simulink model "TransmissionSystem"  (R2026a)
settings: Solver=FixedStepAuto  StopTime=65  FixedStep=0.0005
undefined symbols (not defined in the file or in its folder): f3ea6d5f
settings Model: DataDictionary=ETRS_data.sldd  VariantConfigurationObject=vConfigData  Creator=macec  LastModifiedBy=tstic

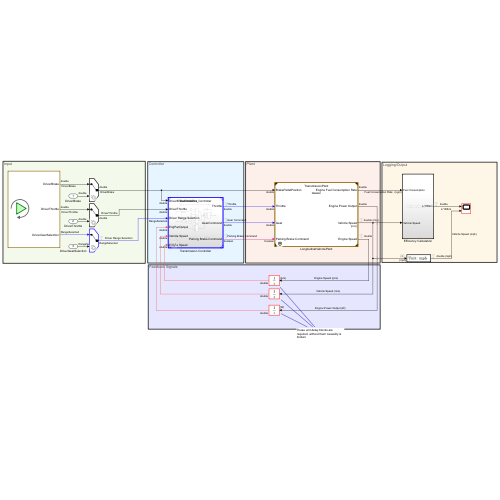
[thumbnail: Simulink's stored preview of the top-level diagram]
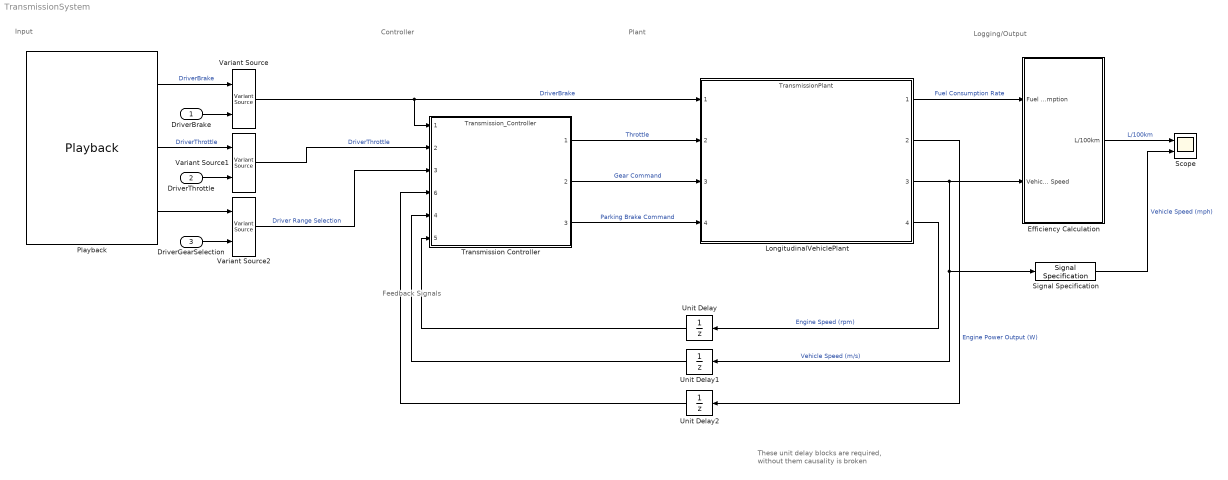
== system TransmissionSystem ==
  note: Logging/Output
  note: These unit delay blocks are required, without them causality is broken
  note: Feedback Signals
  note: Plant
  note: Controller
  note: Input
  DriverBrake : Inport  Interpolate=off
  DriverThrottle : Inport  Port=2  Interpolate=off
  DriverGearSelection : Inport  Port=3  OutDataTypeStr=Enum: RangeSelected  Interpolate=off
  Efficiency Calculation : Subsystem
  LongitudinalVehiclePlant : ModelReference  ModelNameDialog=TransmissionPlant.slxp  ModelReferenceVersion=1.92  CopyOfModelProtected=on  InputSignalHandling=Zero-order hold
  Playback : Playback  NumPorts=3  PartName=f3ea6d5f-6941-4fcc-8b84-64e5b7c9aa8d  TablePosition=Bottom
  Scope : Scope  NumInputPorts=2
  Signal Specification : SignalSpecification  Unit=mph
  Transmission Controller : ModelReference  ModelNameDialog=Transmission_Controller  SimulationMode=Normal  ModelReferenceVersion=1.50
      settings: PortSchema="{\"entries\":[{\"content\":{\"sides\":[{\"content\":{\"connectorIds\":[\"In1\",\"In2\",\"In3\",\"In6\",\"In4\",\"In5\"]},\"type\":\"ConnectorPlacement.EquallySpacedRectSide\",\"uuid\":\"b399a4c7-d8ad-4ca5-9a1c-e50ab35ecd17\"},{\"content\":{\"connectorIds\":[\"Out1\",\"Out2\",\"Out3\"],\"side\":\"RIGHT\"},\"type\":\"ConnectorPlacement.EquallySpacedRectSide\",\"uuid\":\"9df3f294-5faa-4a5a-9200-b853d4fc415e\"},{\"content\":{\"side\":\"TOP\"},\"type\":\"ConnectorPlacement.EquallySpacedRectSide\",\"uuid\":\"c4260467-83a0-4e75-b61d-5877b34bac92\"}]},\"type\":\"ConnectorPlacement.EquallySpacedConnector\",\"uuid\":\"b734fedc-84df-4e62-9d7f-c223df7b0c35\"}],\"packageUris\":[\"http://schema.mathworks.com/mf0/Connector/R2020b\"],\"version\":\"1.0\"}"
  Unit Delay : UnitDelay  SampleTime=-1
  Unit Delay1 : UnitDelay  SampleTime=-1
  Unit Delay2 : UnitDelay  SampleTime=-1
  Variant Source : VariantSource  VariantControls={V == RunType.Simulate, V == RunType.Test}
  Variant Source1 : VariantSource  VariantControls={V == RunType.Simulate, V == RunType.Test}
  Variant Source2 : VariantSource  VariantControls={V == RunType.Simulate, V == RunType.Test}
  wires:
  Variant Source2/1 -> Transmission Controller/3  "Driver Range Selection"
  Transmission Controller/2 -> LongitudinalVehiclePlant/3  "Gear Command"
  Transmission Controller/3 -> LongitudinalVehiclePlant/4  "Parking Brake Command"
  Unit Delay/1 -> Transmission Controller/5
  Unit Delay1/1 -> Transmission Controller/4
  Transmission Controller/1 -> LongitudinalVehiclePlant/2  "Throttle"
  Variant Source/1 -> Transmission Controller/1, LongitudinalVehiclePlant/1  "DriverBrake"
  Variant Source1/1 -> Transmission Controller/2  "DriverThrottle"
  Efficiency Calculation/1(L/100km) -> Scope/1  "L/100km"
  LongitudinalVehiclePlant/4 -> Unit Delay/1  "Engine Speed (rpm)"
  LongitudinalVehiclePlant/3 -> Efficiency Calculation/2(Vehicle Speed), Signal Specification/1, Unit Delay1/1  "Vehicle Speed (m/s)"
  LongitudinalVehiclePlant/1 -> Efficiency Calculation/1(Fuel Consumption)  "Fuel Consumption Rate"
  LongitudinalVehiclePlant/2 -> Unit Delay2/1  "Engine Power Output (W)"
  Playback/1 -> Variant Source/1  "DriverBrake"
  Playback/2 -> Variant Source1/1  "DriverThrottle"
  Playback/3 -> Variant Source2/1
  DriverBrake/1 -> Variant Source/2
  DriverThrottle/1 -> Variant Source1/2
  DriverGearSelection/1 -> Variant Source2/2
  Signal Specification/1 -> Scope/2  "Vehicle Speed (mph)"
  Unit Delay2/1 -> Transmission Controller/6

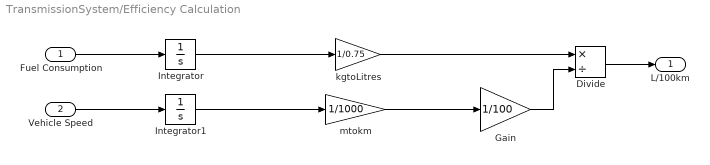
== system TransmissionSystem/Efficiency Calculation ==
  Fuel Consumption : Inport
  Vehicle Speed : Inport  Port=2
  Divide : Product  Inputs=*/
  Gain : Gain  Gain=1/100
  Integrator : Integrator
  Integrator1 : Integrator  InitialCondition=0.0001
  kgtoLitres : Gain  Gain=1/0.75
  mtokm : Gain  Gain=1/1000
  L/100km : Outport
  wires:
  Gain/1 -> Divide/2
  mtokm/1 -> Gain/1
  Vehicle Speed/1 -> Integrator1/1
  Integrator/1 -> kgtoLitres/1
  Integrator1/1 -> mtokm/1
  kgtoLitres/1 -> Divide/1
  Divide/1 -> L/100km/1
  Fuel Consumption/1 -> Integrator/1
